simulink model "mcb_microchip_pmsm_foc_QDEC_SAME54"  (R2023b)
settings: Solver=FixedStepDiscrete  StartTime=0.0  StopTime=6  FixedStep=5e-5  RelTol=1e-3  EnableMultiTasking=on
InitFcn:
  | mcb_microchip_pmsm_foc_QDEC_SAME54_data;
values from neighbouring files (symbols this model uses):
  PI_params = mcb.internal.SetControllerParameters(pmsm,inverter,PU_System,T_pwm,2*Ts,Ts_speed)    [mcb_microchip_pmsm_foc_QDEC_SAME54_data.m]
  PU_System = mcb_SetPUSystem(pmsm,inverter)    [mcb_microchip_pmsm_foc_QDEC_SAME54_data.m]
  PWM_frequency = 20e3    (= 20000)    [mcb_microchip_pmsm_foc_QDEC_SAME54_data.m]
  Ts = T_pwm    (= 5e-05)    [mcb_microchip_pmsm_foc_QDEC_SAME54_data.m]
  Ts_motor = T_pwm    (= 5e-05)    [mcb_microchip_pmsm_foc_QDEC_SAME54_data.m]
  Ts_simulink = T_pwm    (= 5e-05)    [mcb_microchip_pmsm_foc_QDEC_SAME54_data.m]
  Ts_speed = 10 * Ts    (= 0.0005)    [mcb_microchip_pmsm_foc_QDEC_SAME54_data.m]
undefined symbols (not defined in the file or in its folder): AIN0, inverter, PA02, PA03, PA08, PA09, PA10, PA11, PA12, PA13, PA16, PA17, PA18, pad0, pad1, pad2, pad3, PB08, PC16, PC17, PC18, Pin, pmsm, SAME54P20A, Timer, TQFP128, VREFA, wo0, wo1, wo2, wo4, wo5, wo6
libraries: MCHP_Blockset x13, simulink x13, mcbcontrolslib x9, slpidlib x3, mcbpositiondecoderlib x3, mcbplantlib x1, autolibpmsmexterior x1
(part 1 of 4)
settings Model: Creator=Lubin Kerhuel  LastModifiedBy=I69995
settings SolverCC: AlgebraicLoopSolver=TrustRegion
settings DataIOCC: SaveFormat=StructureWithTime  ReturnWorkspaceOutputs=off
settings OptimizationCC: DefaultParameterBehavior=Inlined  DefaultUnderspecifiedDataType=single  EnhancedBackFolding=on  PassReuseOutputArgsAs=Individual arguments  OptimizeBlockOrder=speed  DifferentSizesBufferReuse=on  OptimizationCustomize=off  EfficientTunableParamExpr=on
settings DebuggingCC: MultiTaskDSMMsg=none  ParameterTunabilityLossMsg=error  FcnCallInpInsideContextMsg=warning  UnconnectedInputMsg=warning  UnconnectedOutputMsg=warning  UnconnectedLineMsg=warning  SFExecutionAtInitializationDiag=none  ArithmeticOperatorsInVariantConditions=warning
settings HardwareCC: ProdBitPerPointer=32  ProdBitPerSizeT=32  ProdBitPerPtrDiffT=32  ProdLargestAtomicInteger=Integer  ProdWordSize=32  ProdLongLongMode=on  ProdHWDeviceType=ARM Compatible->ARM Cortex
settings ModelReferenceCC: EnableRefExpFcnMdlSchedulingChecks=on  ModelReferenceNumInstancesAllowed=Single  PropagateSignalLabelsOutOfModel=off
settings SFSimCC: SimUseLocalCustomCode=off  MATLABDynamicMemAlloc=off  CustomCodeUndefinedFunction=UseInterfaceOnly
settings RTWCC: Description=Microchip Embedded Target Cortex M7 (real-time)  SystemTargetFile=MCHP_ARM7_stf.tlc  TemplateMakefile=MCHP_ARM7.tmf  GenerateReport=on  RTWUseLocalCustomCode=off  Toolchain=xc32 - v4.30 for Mirochip SAMx7 device  BuildConfiguration=Specify  IncludeHyperlinkInReport=on  LaunchReport=on  GenerateTraceInfo=on  GenerateTraceReport=on  GenerateTraceReportSl=on  GenerateTraceReportSf=on  GenerateTraceReportEml=on  DLArmComputeVersion=19.05
settings CodeAppCC: ForceParamTrailComments=on  IgnoreCustomStorageClasses=off  MaxIdLength=255  OperatorAnnotations=on  SimulinkDataObjDesc=on  SFDataObjDesc=on  InsertBlockDesc=on  InternalIdentifier=Classic
settings STFCustomTargetCC: TargetLangStandard=C89/C90 (ANSI)  MultiwordLength=256  IncludeMdlTerminateFcn=off  CombineOutputUpdateFcns=on  CombineSignalStateStructs=on  SuppressErrorStatus=on  ERTCustomFileBanners=on  SupportContinuousTime=off  RemoveResetFunc=on  MATLABClassNameForMDSCustomization=Simulink.SoftwareTarget.ERTCustomization  UseToolchainInfoCompliant=on  SystemTargetFile=MCHP_ARM7_stf.tlc
settings ERTTargetCC: ParMdlRefBuildCompliant=off  CompOptLevelCompliant=off  ConcurrentExecutionCompliant=off  IncludeMdlTerminateFcn=off  CombineSignalStateStructs=on  SuppressErrorStatus=on  SupportNonInlinedSFcns=on  ModelStepFunctionPrototypeControlCompliant=off  CPPClassGenCompliant=off  ExtModeStaticAllocSize=2000  InlinedParameterPlacement=NonHierarchical  ERTSrcFileBannerTemplate=MCHP_dsPIC_code_template.cgt  ERTHdrFileBannerTemplate=MCHP_dsPIC_code_template.cgt  ERTDataSrcFileTemplate=MCHP_dsPIC_code_template.cgt  ERTDataHdrFileTemplate=MCHP_dsPIC_code_template.cgt  ERTCustomFileTemplate=MCHP_main.tlc

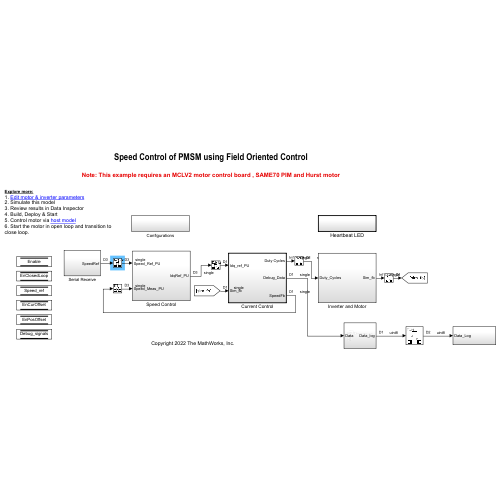
[thumbnail: Simulink's stored preview of the top-level diagram]
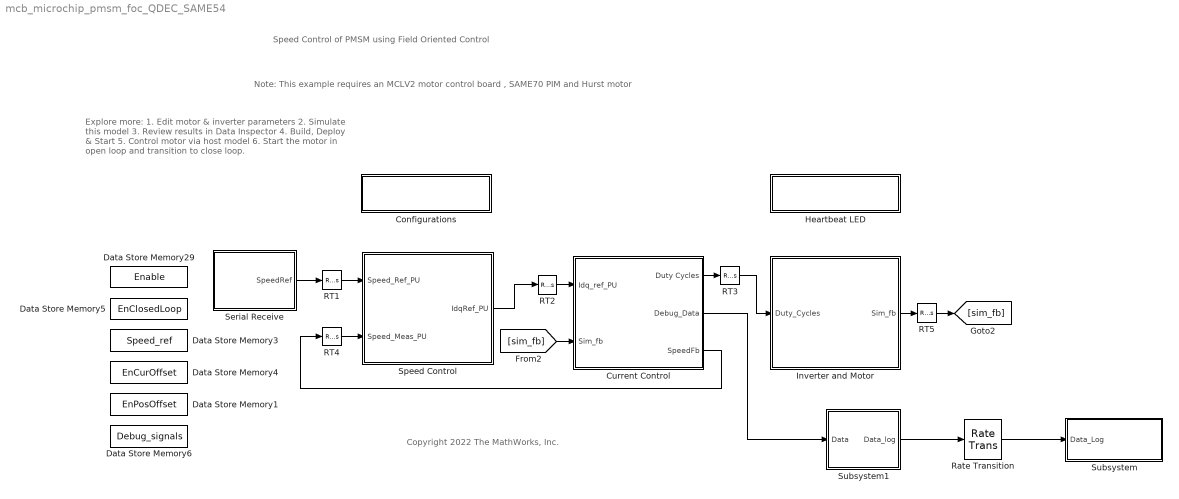
== system mcb_microchip_pmsm_foc_QDEC_SAME54 ==
  note: Note: This example requires an MCLV2 motor control board , SAME70 PIM and Hurst motor
  note: Copyright 2022 The MathWorks, Inc.
  note: Speed Control of PMSM using Field Oriented Control
  note: Explore more:
      | 1. Edit motor & inverter parameters
      | 2. Simulate this model
      | 3. Review results in Data Inspector
      | 4. Build, Deploy & Start
      | 5. Control motor via host model
      | 6. Start the motor in open loop and transition to close loop.
  Configurations : Subsystem
  Current Control : Subsystem  TreatAsAtomicUnit=on
  Data Store Memory1 : DataStoreMemory  DataStoreName=EnPosOffset  ShowAdditionalParam=off  OutDataTypeStr=boolean
  Data Store Memory29 : DataStoreMemory  DataStoreName=Enable  ReadBeforeWriteMsg=warning  WriteAfterWriteMsg=warning  WriteAfterReadMsg=warning  InitialValue=1  ShowAdditionalParam=off  OutDataTypeStr=boolean
  Data Store Memory3 : DataStoreMemory  DataStoreName=Speed_ref  ReadBeforeWriteMsg=warning  WriteAfterWriteMsg=warning  WriteAfterReadMsg=warning  InitialValue=0.1  ShowAdditionalParam=off  OutDataTypeStr=dataType
  Data Store Memory4 : DataStoreMemory  DataStoreName=EnCurOffset  ReadBeforeWriteMsg=warning  WriteAfterWriteMsg=warning  WriteAfterReadMsg=warning  ShowAdditionalParam=off  OutDataTypeStr=boolean
  Data Store Memory5 : DataStoreMemory  DataStoreName=EnClosedLoop  ReadBeforeWriteMsg=warning  WriteAfterWriteMsg=warning  WriteAfterReadMsg=warning  ShowAdditionalParam=off  OutDataTypeStr=boolean
  Data Store Memory6 : DataStoreMemory  DataStoreName=Debug_signals  ReadBeforeWriteMsg=warning  WriteAfterWriteMsg=warning  WriteAfterReadMsg=warning  InitialValue=5  ShowAdditionalParam=off  OutDataTypeStr=uint16
  Heartbeat LED : Subsystem  TreatAsAtomicUnit=on
  Inverter and Motor : Subsystem
  RT1 : RateTransition  Deterministic=off  OutPortSampleTime=Ts_speed
  RT2 : RateTransition  Deterministic=off
  RT3 : RateTransition  Deterministic=off
  RT4 : RateTransition  Deterministic=off  OutPortSampleTime=Ts_speed
  RT5 : RateTransition  Deterministic=off
  Rate Transition : RateTransition  OutPortSampleTime=Ts_SerialCom
  Serial Receive : Subsystem
  Speed Control : Subsystem  SystemSampleTime=Ts_speed
  Subsystem : Subsystem
  Subsystem1 : Subsystem
  wires:
  RT5/1 -> [sim_fb]
  [sim_fb] -> Current Control/2(Sim_fb)
  Inverter and Motor/1(Sim_fb) -> RT5/1
  RT3/1 -> Inverter and Motor/1(Duty_Cycles)
  Speed Control/1(IdqRef_PU) -> RT2/1
  RT4/1 -> Speed Control/2(Speed_Meas_PU)
  RT2/1 -> Current Control/1(Idq_ref_PU)
  Current Control/3(SpeedFb) -> RT4/1
  Current Control/1(Duty Cycles) -> RT3/1
  Serial Receive/1(SpeedRef) -> RT1/1
  RT1/1 -> Speed Control/1(Speed_Ref_PU)
  Subsystem1/1(Data_log) -> Rate Transition/1
  Current Control/2(Debug_Data) -> Subsystem1/1(Data)
  Rate Transition/1 -> Subsystem/1(Data_Log)
